simulink model "autopilot_total"  (R2021b)
settings: Solver=ode4  StartTime=0.0  StopTime=T  FixedStep=P.Ts  RelTol=1e-6  AbsTol=1e-3  EnableMultiTasking=on
values from neighbouring files (symbols this model uses):
  k_VI = 0.8    [forces_moments_testing.m]
  k_VP = 0.5    [forces_moments_testing.m]
undefined symbols (not defined in the file or in its folder): forces_moments, P, true_states
libraries: simulink x3
settings Model: Creator=beard  LastModifiedBy=joaomoura
settings SolverCC: AutoScaleAbsTol=off  AlgebraicLoopSolver=TrustRegion
settings DataIOCC: LimitDataPoints=on  SaveFormat=Array  ReturnWorkspaceOutputs=off
settings OptimizationCC: ExpressionDepthLimit=2147483647  InitFltsAndDblsToZero=on  LifeSpan=inf
settings DebuggingCC: UnderspecifiedInitializationDetection=Classic  MergeDetectMultiDrivingBlocksExec=none  SolverPrmCheckMsg=warning  FcnCallInpInsideContextMsg=warning  StateNameClashWarn=warning  PregeneratedLibrarySubsystemCodeDiagnostic=none  SFUnexpectedBacktrackingDiag=warning  SFNoUnconditionalDefaultTransitionDiag=warning  SFExecutionAtInitializationDiag=none  SFMachineParentedDataDiag=warning  ArithmeticOperatorsInVariantConditions=warning
settings HardwareCC: ProdBitPerPointer=32  ProdBitPerSizeT=32  ProdBitPerPtrDiffT=32  ProdLargestAtomicFloat=None  ProdIntDivRoundTo=Undefined  ProdEndianess=Unspecified  ProdWordSize=32  ProdHWDeviceType=32-bit Generic
settings ModelReferenceCC: PropagateSignalLabelsOutOfModel=off
settings SFSimCC: SimUseLocalCustomCode=off  CustomCodeUndefinedFunction=UseInterfaceOnly
settings RTWCC: RTWUseLocalCustomCode=off
settings CodeAppCC: StateflowObjectComments=on
settings GRTTargetCC: TargetLangStandard=C89/C90 (ANSI)  CombineOutputUpdateFcns=off  GRTInterface=on
settings ConfigComp: CovMetricSettings=dw  CovSaveCumulativeToWorkspaceVar=on  CovSaveSingleToWorkspaceVar=on  CovExternalEMLEnable=off  CovSFcnEnable=off

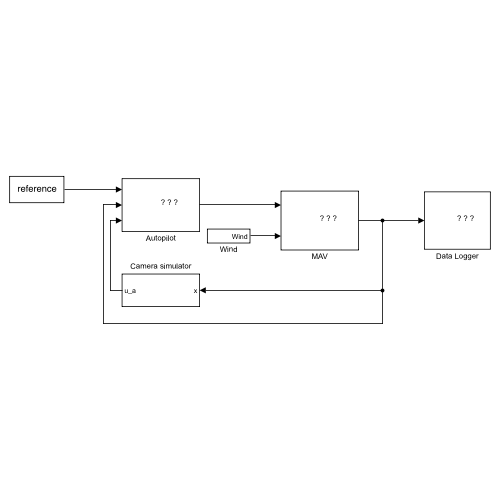
[thumbnail: Simulink's stored preview of the top-level diagram]
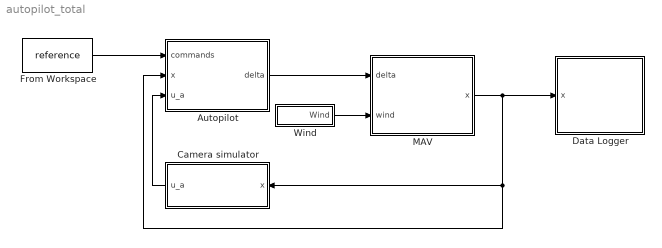
== system autopilot_total ==
  Autopilot : Subsystem
      mask Display: image(imread('simulink_imgs/kestrel.jpg'))
  Camera simulator : Subsystem
  Data Logger : Subsystem
      mask Display: image(imread('simulink_imgs/data_logger.png'))
  From Workspace : FromWorkspace  VariableName=reference
  MAV : Subsystem
      mask Display: image(imread('simulink_imgs/batcam.png'))
  Wind : Subsystem
  wires:
  Wind/1(Wind) -> MAV/2(wind)
  MAV/1(x) -> Camera simulator/1(x), Autopilot/2(x), Data Logger/1(x)
  Autopilot/1(delta) -> MAV/1(delta)
  From Workspace/1 -> Autopilot/1(commands)
  Camera simulator/1(u_a) -> Autopilot/3(u_a)

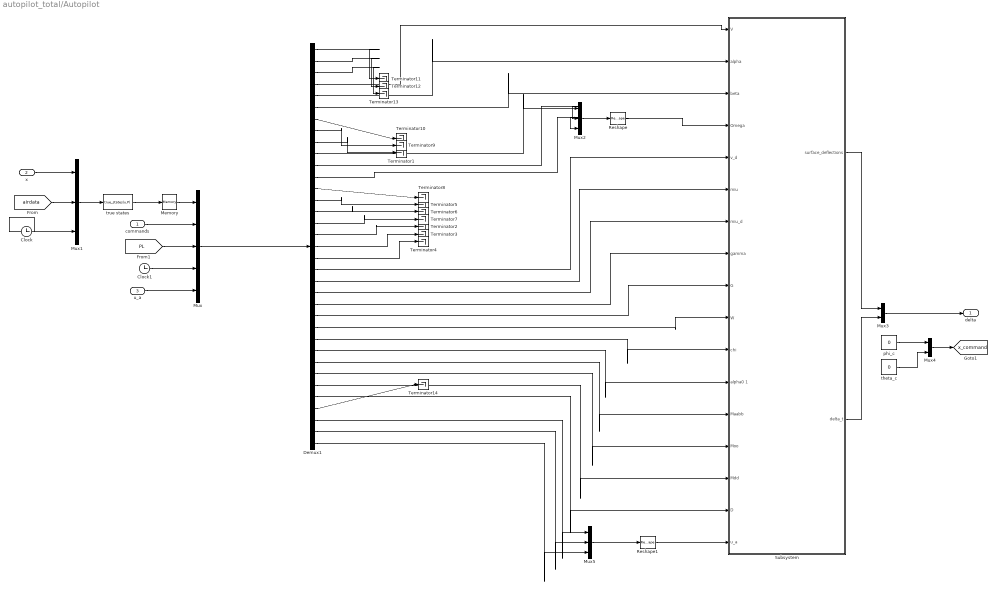
== system autopilot_total/Autopilot ==
  commands : Inport
  x : Inport  Port=2
  u_a : Inport  Port=3
  Clock : Clock
  Clock1 : Clock
  Demux1 : Demux  Outputs=19+1+11+1+3
  Memory : Memory
  Mux : Mux  Inputs=5
  Mux1 : Mux  Inputs=3
  Mux2 : Mux  Inputs=3
  Mux3 : Mux  Inputs=2
  Mux4 : Mux  Inputs=2
  Mux5 : Mux  Inputs=3
  Reshape : Reshape  OutputDimensionality=Customize  OutputDimensions=[3,1]
  Reshape1 : Reshape  OutputDimensionality=Customize  OutputDimensions=[3,1]
  Subsystem : Subsystem
  Terminator{1..14} (14 alike) : Terminator
  phi_c : Constant  Value=0
  theta_c : Constant  Value=0
  true states : MATLABFcn  MATLABFcn=true_states(u,P)  OutputDimensions=19  SampleTime=P.Ts
  delta : Outport  VectorParamsAs1DForOutWhenUnconnected=off
  tag scope: x_command=global
  wires:
  Clock/1 -> Mux1/3
  Mux3/1 -> delta/1
  Mux4/1 -> [x_command]
  commands/1 -> Mux/2
  Mux1/1 -> true states/1
  x/1 -> Mux1/1
  true states/1 -> Memory/1
  [airdata] -> Mux1/2
  Memory/1 -> Mux/1
  Clock1/1 -> Mux/4
  [PL] -> Mux/3
  Mux/1 -> Demux1/1
  Demux1/4 -> Subsystem/1(V)
  Demux1/5 -> Subsystem/2(alpha)
  Demux1/6 -> Subsystem/3(beta)
  Demux1/20 -> Subsystem/5(v_d)
  Demux1/10 -> Mux2/1
  Demux1/11 -> Mux2/2
  Demux1/12 -> Mux2/3
  Mux2/1 -> Reshape/1
  Demux1/21 -> Subsystem/6(miu)
  Demux1/22 -> Subsystem/7(miu_d)
  Demux1/23 -> Subsystem/8(gamma)
  Demux1/24 -> Subsystem/9(G)
  Demux1/25 -> Subsystem/10(W)
  u_a/1 -> Mux/5
  Demux1/26 -> Subsystem/11(chi)
  Demux1/27 -> Subsystem/12(alpha0 1)
  Demux1/28 -> Subsystem/13(Maabb)
  Demux1/29 -> Subsystem/14(Moo)
  Demux1/30 -> Subsystem/15(Mdd)
  Demux1/19 -> Terminator4/1
  Demux1/18 -> Terminator3/1
  Demux1/17 -> Terminator2/1
  Demux1/16 -> Terminator7/1
  Demux1/15 -> Terminator6/1
  Demux1/14 -> Terminator5/1
  Demux1/13 -> Terminator8/1
  Demux1/9 -> Terminator1/1
  Demux1/8 -> Terminator9/1
  Demux1/7 -> Terminator10/1
  Demux1/3 -> Terminator13/1
  Demux1/2 -> Terminator12/1
  Demux1/1 -> Terminator11/1
  Subsystem/1(surface_deflections) -> Mux3/1
  Subsystem/2("delta_t ") -> Mux3/2
  phi_c/1 -> Mux4/1
  theta_c/1 -> Mux4/2
  Demux1/31 -> Subsystem/16(D)
  Demux1/32 -> Terminator14/1
  Reshape/1 -> Subsystem/4("Omega ")
  Demux1/33 -> Mux5/1
  Demux1/34 -> Mux5/2
  Demux1/35 -> Mux5/3
  Mux5/1 -> Reshape1/1
  Reshape1/1 -> Subsystem/17(u_a)

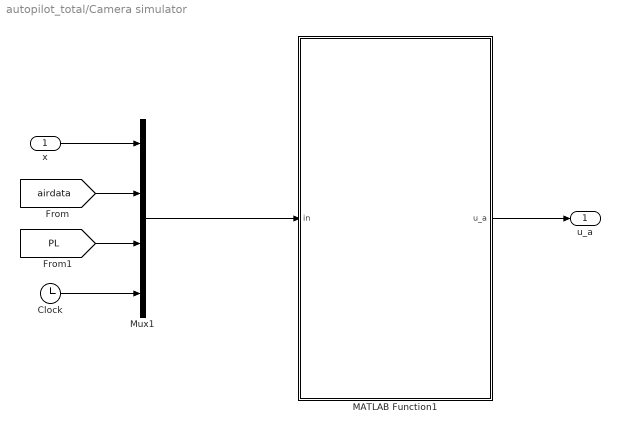
== system autopilot_total/Camera simulator ==
  x : Inport
  Clock : Clock
  MATLAB Function1 : MATLAB Function  TreatAsAtomicUnit=on
  Mux1 : Mux
  u_a : Outport
  wires:
  MATLAB Function1/1(u_a) -> u_a/1
  Clock/1 -> Mux1/4
  [airdata] -> Mux1/2
  [PL] -> Mux1/3
  Mux1/1 -> MATLAB Function1/1(in)
  x/1 -> Mux1/1

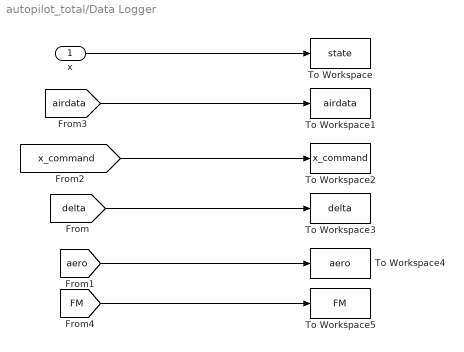
== system autopilot_total/Data Logger ==
  x : Inport
  To Workspace : ToWorkspace  VariableName=state  SaveFormat=Structure With Time  SampleTime=-1
  To Workspace1 : ToWorkspace  VariableName=airdata  SaveFormat=Structure With Time  SampleTime=-1
  To Workspace2 : ToWorkspace  VariableName=x_command  SaveFormat=Structure With Time  SampleTime=-1
  To Workspace3 : ToWorkspace  VariableName=delta  SaveFormat=Structure With Time  SampleTime=-1
  To Workspace4 : ToWorkspace  VariableName=aero  SaveFormat=Structure With Time  SampleTime=-1
  To Workspace5 : ToWorkspace  VariableName=FM  SaveFormat=Structure With Time  SampleTime=-1
  wires:
  x/1 -> To Workspace/1
  [x_command] -> To Workspace2/1
  [delta] -> To Workspace3/1
  [airdata] -> To Workspace1/1
  [aero] -> To Workspace4/1
  [FM] -> To Workspace5/1

== system autopilot_total/MAV ==
  note: Forces & Moments
  note: States
  delta : Inport
  wind : Inport  Port=2
  Dynamics : S-Function  FunctionName=mav_dynamics  Parameters=P  SFunctionDeploymentMode=off  EnableBusSupport=off
  Forces & Moments : Subsystem
  x : Outport  VectorParamsAs1DForOutWhenUnconnected=off
  tag scope: PL=global, airdata=global
  wires:
  Dynamics/1 -> Forces & Moments/1(x), x/1
  Forces & Moments/1("[F M]") -> Dynamics/1
  Forces & Moments/2(air data) -> [airdata]
  delta/1 -> Forces & Moments/2(delta)
  wind/1 -> Forces & Moments/3(wind)
  Forces & Moments/3(PL) -> [PL]

== system autopilot_total/Wind ==
  Constant2 : Constant  Value=[P.wind_n; P.wind_e; P.wind_d]
  Mux1 : Mux  Inputs=2
  Wind Gusts : Subsystem
  Wind : Outport  VectorParamsAs1DForOutWhenUnconnected=off
  wires:
  Constant2/1 -> Mux1/1
  Mux1/1 -> Wind/1
  Wind Gusts/1(gusts) -> Mux1/2

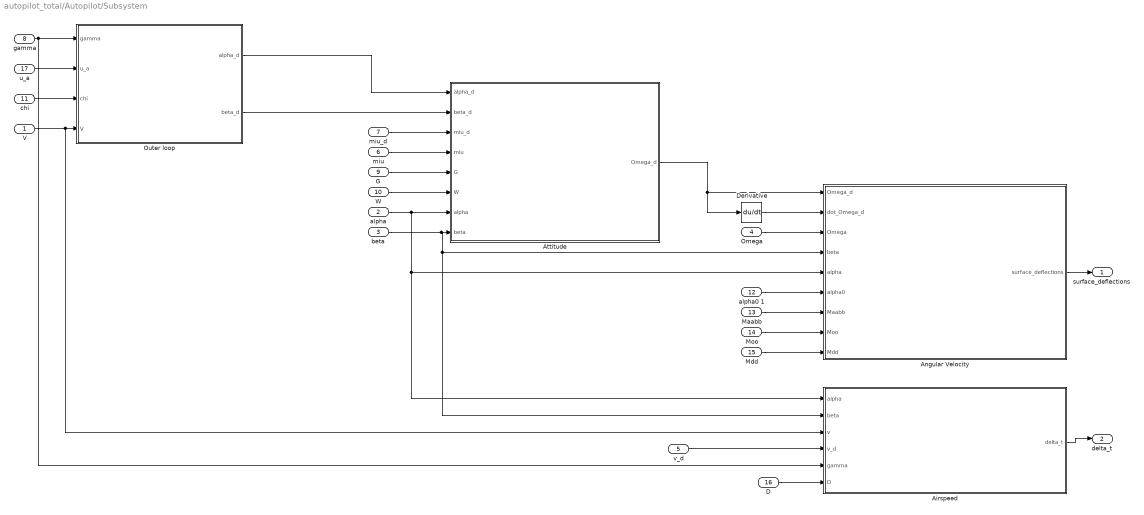
== system autopilot_total/Autopilot/Subsystem ==
  V : Inport
  alpha : Inport  Port=2
  beta : Inport  Port=3
  "Omega " : Inport  Port=4
  v_d : Inport  Port=5
  miu : Inport  Port=6
  miu_d : Inport  Port=7
  gamma : Inport  Port=8
  G : Inport  Port=9
  W : Inport  Port=10
  chi : Inport  Port=11
  alpha0 1 : Inport  Port=12
  Maabb : Inport  Port=13
  Moo : Inport  Port=14
  Mdd : Inport  Port=15
  D : Inport  Port=16
  u_a : Inport  Port=17
  Airspeed : Subsystem
  Angular Velocity : Subsystem
  Attitude : Subsystem
  Derivative : Derivative
  Outer loop : Subsystem
  surface_deflections : Outport  VectorParamsAs1DForOutWhenUnconnected=off
  "delta_t " : Outport  Port=2  VectorParamsAs1DForOutWhenUnconnected=off
  wires:
  Attitude/1(Omega_d) -> Derivative/1, Angular Velocity/1(Omega_d)
  Outer loop/2(beta_d) -> Attitude/2(beta_d)
  v_d/1 -> Airspeed/4(v_d)
  gamma/1 -> Outer loop/1(gamma), Airspeed/5(gamma)
  Airspeed/1("delta_t ") -> "delta_t "/1
  "Omega "/1 -> Angular Velocity/3(Omega)
  miu/1 -> Attitude/4(miu)
  beta/1 -> Airspeed/2(beta), Angular Velocity/4(beta), Attitude/8(beta)
  miu_d/1 -> Attitude/3(miu_d)
  Outer loop/1(alpha_d) -> Attitude/1(alpha_d)
  V/1 -> Outer loop/4(V), Airspeed/3("v ")
  Angular Velocity/1(surface_deflections) -> surface_deflections/1
  alpha/1 -> Attitude/7(alpha), Airspeed/1(alpha), Angular Velocity/5(alpha)
  u_a/1 -> Outer loop/2(u_a)
  chi/1 -> Outer loop/3(chi)
  Derivative/1 -> Angular Velocity/2(dot_Omega_d)
  G/1 -> Attitude/5(G)
  W/1 -> Attitude/6(W)
  alpha0 1/1 -> Angular Velocity/6(alpha0)
  Maabb/1 -> Angular Velocity/7(Maabb)
  Moo/1 -> Angular Velocity/8(Moo)
  Mdd/1 -> Angular Velocity/9(Mdd)
  D/1 -> Airspeed/6(D)

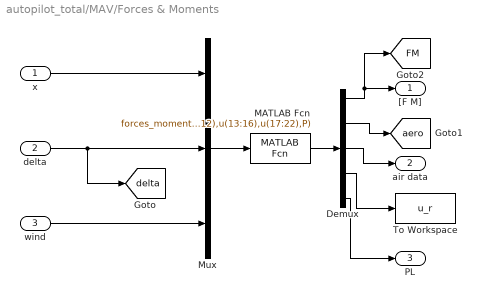
== system autopilot_total/MAV/Forces & Moments ==
  x : Inport
  delta : Inport  Port=2
  wind : Inport  Port=3
  Demux : Demux  Outputs=[6;6;6;1;11]
  MATLAB Fcn : MATLABFcn  MATLABFcn=forces_moments(u(1:12),u(13:16),u(17:22),P)  OutputDimensions=30
  Mux : Mux  Inputs=3
  To Workspace : ToWorkspace  VariableName=u_r  SampleTime=-1
  "[F M]" : Outport  VectorParamsAs1DForOutWhenUnconnected=off
  air data : Outport  Port=2  VectorParamsAs1DForOutWhenUnconnected=off
  PL : Outport  Port=3  VectorParamsAs1DForOutWhenUnconnected=off
  tag scope: FM=global, aero=global, delta=global
  wires:
  Mux/1 -> MATLAB Fcn/1
  Demux/1 -> [FM], "[F M]"/1
  MATLAB Fcn/1 -> Demux/1
  wind/1 -> Mux/3
  delta/1 -> Mux/2, [delta]
  x/1 -> Mux/1
  Demux/3 -> air data/1
  Demux/2 -> [aero]
  Demux/4 -> To Workspace/1
  Demux/5 -> PL/1

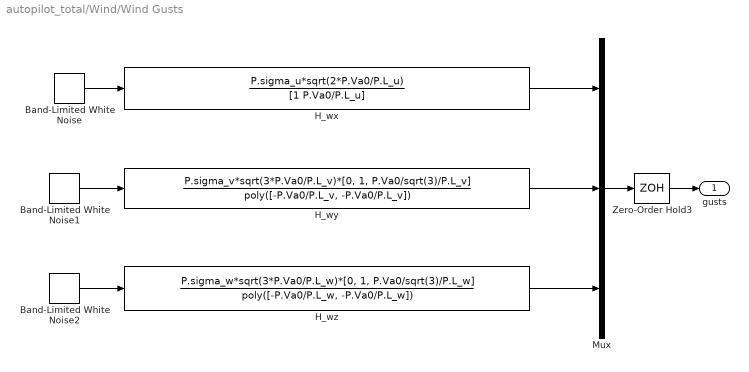
== system autopilot_total/Wind/Wind Gusts ==
  Band-Limited White Noise : simulink/Sources/Band-Limited White Noise  Cov=[1]  Ts=P.Ts  seed=[23341]
  Band-Limited White Noise1 : simulink/Sources/Band-Limited White Noise  Cov=[1]  Ts=P.Ts  seed=[23341]
  Band-Limited White Noise2 : simulink/Sources/Band-Limited White Noise  Cov=[1]  Ts=P.Ts  seed=[23341]
  H_wx : TransferFcn  Numerator=P.sigma_u*sqrt(2*P.Va0/P.L_u)  Denominator=[1 P.Va0/P.L_u]
  H_wy : TransferFcn  Numerator=P.sigma_v*sqrt(3*P.Va0/P.L_v)*[0, 1, P.Va0/sqrt(3)/P.L_v]  Denominator=poly([-P.Va0/P.L_v, -P.Va0/P.L_v])
  H_wz : TransferFcn  Numerator=P.sigma_w*sqrt(3*P.Va0/P.L_w)*[0, 1, P.Va0/sqrt(3)/P.L_w]  Denominator=poly([-P.Va0/P.L_w, -P.Va0/P.L_w])
  Mux : Mux  Inputs=3
  Zero-Order Hold3 : ZeroOrderHold  SampleTime=P.Ts
  gusts : Outport  VectorParamsAs1DForOutWhenUnconnected=off
  wires:
  H_wx/1 -> Mux/1
  Band-Limited White Noise/1 -> H_wx/1
  H_wy/1 -> Mux/2
  Band-Limited White Noise1/1 -> H_wy/1
  H_wz/1 -> Mux/3
  Band-Limited White Noise2/1 -> H_wz/1
  Mux/1 -> Zero-Order Hold3/1
  Zero-Order Hold3/1 -> gusts/1

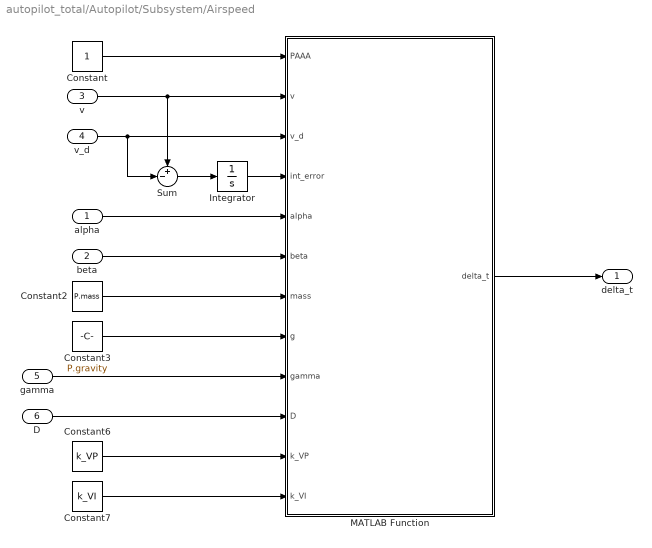
== system autopilot_total/Autopilot/Subsystem/Airspeed ==
  alpha : Inport
  beta : Inport  Port=2
  "v " : Inport  Port=3
  v_d : Inport  Port=4
  gamma : Inport  Port=5
  D : Inport  Port=6
  Constant : Constant
  Constant2 : Constant  Value=P.mass
  Constant3 : Constant  Value=P.gravity
  Constant6 : Constant  Value=k_VP
  Constant7 : Constant  Value=k_VI
  Integrator : Integrator
  MATLAB Function : MATLAB Function  TreatAsAtomicUnit=on
  Sum : Sum  Inputs=+-|
  "delta_t " : Outport  VectorParamsAs1DForOutWhenUnconnected=off
  wires:
  Constant3/1 -> MATLAB Function/8(g)
  gamma/1 -> MATLAB Function/9(gamma)
  Constant7/1 -> MATLAB Function/12(k_VI)
  beta/1 -> MATLAB Function/6(beta)
  Constant6/1 -> MATLAB Function/11(k_VP)
  MATLAB Function/1(delta_t) -> "delta_t "/1
  "v "/1 -> Sum/1, MATLAB Function/2(v)
  Integrator/1 -> MATLAB Function/4(int_error)
  alpha/1 -> MATLAB Function/5(alpha)
  Sum/1 -> Integrator/1
  Constant2/1 -> MATLAB Function/7(mass)
  Constant/1 -> MATLAB Function/1(PAAA)
  v_d/1 -> Sum/2, MATLAB Function/3(v_d)
  D/1 -> MATLAB Function/10(D)

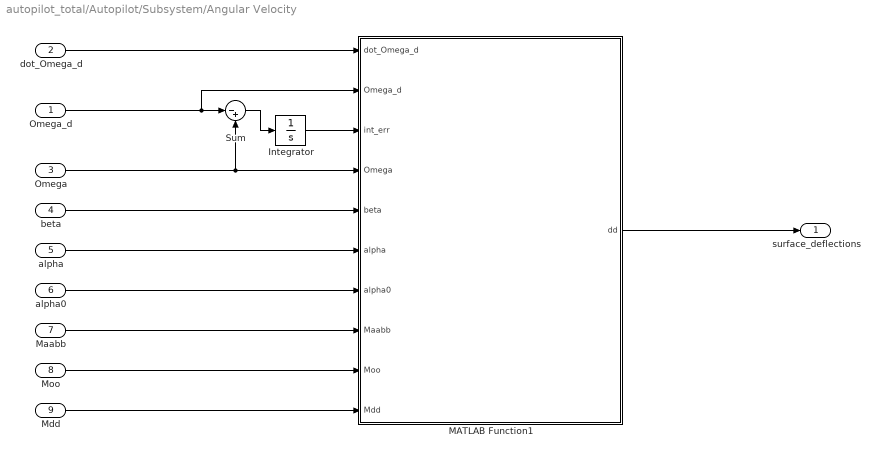
== system autopilot_total/Autopilot/Subsystem/Angular Velocity ==
  Omega_d : Inport
  dot_Omega_d : Inport  Port=2
  Omega : Inport  Port=3
  beta : Inport  Port=4
  alpha : Inport  Port=5
  alpha0 : Inport  Port=6
  Maabb : Inport  Port=7
  Moo : Inport  Port=8
  Mdd : Inport  Port=9
  Integrator : Integrator
  MATLAB Function1 : MATLAB Function  TreatAsAtomicUnit=on
  Sum : Sum  Inputs=|-+
  surface_deflections : Outport  VectorParamsAs1DForOutWhenUnconnected=off
  wires:
  Maabb/1 -> MATLAB Function1/8(Maabb)
  Omega_d/1 -> MATLAB Function1/2(Omega_d), Sum/1
  Sum/1 -> Integrator/1
  Mdd/1 -> MATLAB Function1/10(Mdd)
  dot_Omega_d/1 -> MATLAB Function1/1(dot_Omega_d)
  beta/1 -> MATLAB Function1/5(beta)
  Omega/1 -> Sum/2, MATLAB Function1/4(Omega)
  Moo/1 -> MATLAB Function1/9(Moo)
  alpha0/1 -> MATLAB Function1/7(alpha0)
  Integrator/1 -> MATLAB Function1/3(int_err)
  MATLAB Function1/1(dd) -> surface_deflections/1
  alpha/1 -> MATLAB Function1/6(alpha)

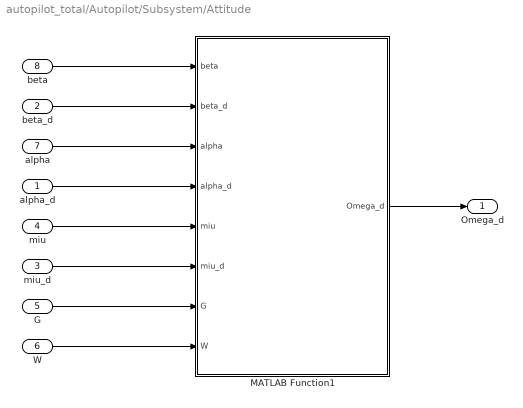
== system autopilot_total/Autopilot/Subsystem/Attitude ==
  alpha_d : Inport
  beta_d : Inport  Port=2
  miu_d : Inport  Port=3
  miu : Inport  Port=4
  G : Inport  Port=5
  W : Inport  Port=6
  alpha : Inport  Port=7
  beta : Inport  Port=8
  MATLAB Function1 : MATLAB Function  TreatAsAtomicUnit=on
  Omega_d : Outport  VectorParamsAs1DForOutWhenUnconnected=off
  wires:
  MATLAB Function1/1(Omega_d) -> Omega_d/1
  alpha_d/1 -> MATLAB Function1/4(alpha_d)
  beta_d/1 -> MATLAB Function1/2(beta_d)
  miu_d/1 -> MATLAB Function1/6(miu_d)
  miu/1 -> MATLAB Function1/5(miu)
  beta/1 -> MATLAB Function1/1(beta)
  alpha/1 -> MATLAB Function1/3(alpha)
  G/1 -> MATLAB Function1/7(G)
  W/1 -> MATLAB Function1/8(W)

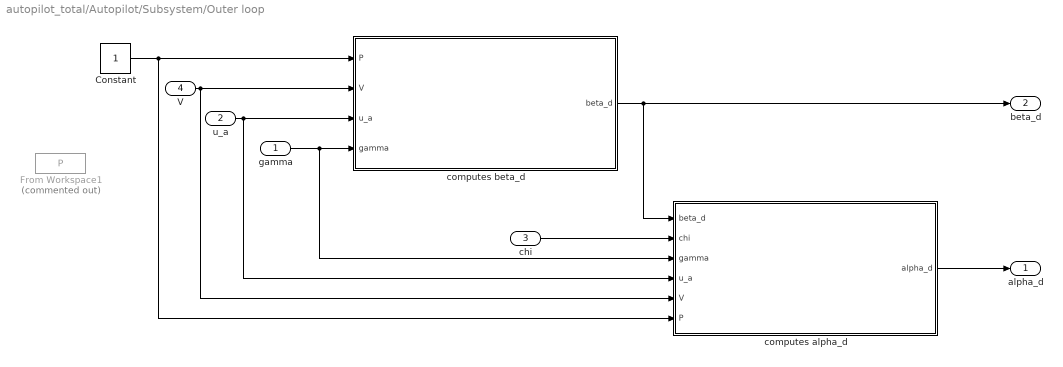
== system autopilot_total/Autopilot/Subsystem/Outer loop ==
  gamma : Inport
  u_a : Inport  Port=2
  chi : Inport  Port=3
  V : Inport  Port=4
  Constant : Constant
  From Workspace1 : FromWorkspace  Commented=on  VariableName=P
  computes alpha_d : Subsystem
  computes beta_d : Subsystem
  alpha_d : Outport
  beta_d : Outport  Port=2
  wires:
  computes beta_d/1(beta_d) -> computes alpha_d/1(beta_d), beta_d/1
  computes alpha_d/1(alpha_d) -> alpha_d/1
  gamma/1 -> computes alpha_d/3(gamma), computes beta_d/4(gamma)
  u_a/1 -> computes beta_d/3(u_a), computes alpha_d/4(u_a)
  chi/1 -> computes alpha_d/2(chi)
  Constant/1 -> computes alpha_d/6(P), computes beta_d/1(P)
  V/1 -> computes beta_d/2(V), computes alpha_d/5(V)

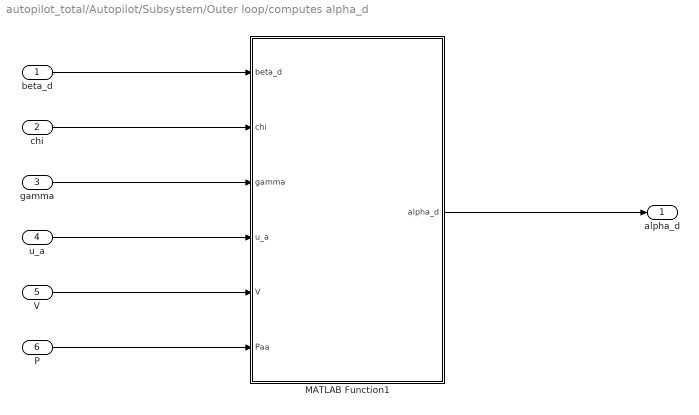
== system autopilot_total/Autopilot/Subsystem/Outer loop/computes alpha_d ==
  beta_d : Inport
  chi : Inport  Port=2
  gamma : Inport  Port=3
  u_a : Inport  Port=4
  V : Inport  Port=5
  P : Inport  Port=6
  MATLAB Function1 : MATLAB Function  TreatAsAtomicUnit=on
  alpha_d : Outport  VectorParamsAs1DForOutWhenUnconnected=off
  wires:
  MATLAB Function1/1(alpha_d) -> alpha_d/1
  beta_d/1 -> MATLAB Function1/1(beta_d)
  P/1 -> MATLAB Function1/6(Paa)
  u_a/1 -> MATLAB Function1/4(u_a)
  chi/1 -> MATLAB Function1/2(chi)
  gamma/1 -> MATLAB Function1/3(gamma)
  V/1 -> MATLAB Function1/5(V)

== system autopilot_total/Autopilot/Subsystem/Outer loop/computes beta_d ==
  P : Inport
  V : Inport  Port=2
  u_a : Inport  Port=3
  gamma : Inport  Port=4
  MATLAB Function1 : MATLAB Function  TreatAsAtomicUnit=on
  beta_d : Outport  VectorParamsAs1DForOutWhenUnconnected=off
  wires:
  MATLAB Function1/1(beta_d) -> beta_d/1
  P/1 -> MATLAB Function1/1(Paa)
  u_a/1 -> MATLAB Function1/3(u_a)
  gamma/1 -> MATLAB Function1/4(gamma)
  V/1 -> MATLAB Function1/2(V)

== matlab function autopilot_total/Autopilot/Subsystem/Outer loop/computes beta_d/MATLAB Function1 ==
  data: Paa input; V input; u_a input; gamma input; beta_d output
function beta_d = controller(Paa,V,u_a,gamma)
    P.mass = 25;
    P.rho = 1.2682;
    P.gravity = 9.8000;
    P.C_Y_beta = -0.9800;
    P.S_wing = 0.5500;
    
    % params
    q_bar = 0.5*P.rho*V^2;
    
    % control law

    beta_d = ([0;0;1]'*u_a*cos(gamma)) / (q_bar*P.S_wing*P.C_Y_beta - P.mass*P.gravity*sin(gamma));

end

== matlab function autopilot_total/Camera simulator/MATLAB Function1 ==
  data: in input; u_a output
% function u_a = ua(in)
%     % params
%     % vw is wind
%     
%     V = in(13);  
%     v = in(4,5,6); 
%     vw = [in(14,15),0];
% 
%     k1 = 1;
%     k3 = 5;
%     k4 = 3.5;
%     m = 25;
%     q = [1, 0, 0]; % Centroid                   %é só isto?
%     u = [0, 0 , 1]; % Direction of the lines    % duas vezes os mesmo u?
%     u = transpose([1, 0, 0]);
%     rho = transpose([0, 1, 0]);
%     n = transpose([0, 0, 1]);
%     delta1 = transpose(n)*q;
%     vwy = transpose(rho)*vw;
%     vdy = -k1*delta1 - vwy;
%     v = transpose(rho)*v;
%     d = -n*(v + vw);
%     w_star = 0.4; % desired translational optical flow in the direction n.
%     w = (v +vw)/d; 
%     vy = v(2);  % vy = transpose(rho)*
%     delta3 = vy - vdy;
%     % control law
% 
%     u_a = (m*V) / (transpose(v)*u)*(k1*k3*delta3*n-k4*(transpose(n)*w-w_star)*rho);
% 
% end

%function u_a = ua(n,rho, cam,points1,points2, vel, m, V, wind,u,k1,k3,k4, R)
%function u_a = ua(pos, vel, V, wind)
function u_a = ua(in)
    % assume cam = [x, y, z] where x, y and z are measured in relation to L
    % (0, 0 ,0) is the position of the camera assumed in the center of mass
    % of the aircraft
    % points1 - array with points of the left line
    % points2 - array with points of the right line
    % in this code it is assumed the points come in the following format:
    % points1 = [-5,0,0, -5,5,0, -5,10,0, -5,15,0]; % line on the left
    % wind = [wx, wy, wz]     
    % vel = [vx, vy, vz] of the plane relative to the wind
    % V the velocity of the aircraft
    % k1, k3 and k4 are gain values
    % m the mass
    % R is the rotation matrix
    L = [0,0,0];


    pos = [in(1),in(2),in(3)]';
    vel = [in(4),in(5),in(6)]';
    V = in(13);  
    wind = [in(14),in(15),0]';

    cam = [pos(1)- L(1), pos(2)- L(2), (-pos(3)) - L(3)]; %pos of aircraft relative to L


    k1 = 1;
    k3 = 5;
    k4 = 3.5;
    mass = 25;

    n = [0, 0, 1]';
    rho = [0, 1, 0]';
    u = [1, 0, 0]';

    points1 = [-5,0,0, -5,5,0, -5,10,0, -5,15,0];
    points2 = [5,0,0, 5,5,0, 5,10,0, 5,15,0];
    
    R = rotx(10);  %o que é aqui??

    P1 = reshape(points1, 3, floor(length(points1)/3))';
     % Assuming an ideal spherical camera
    q = [0 0 0];
    for i=1:floor(length(points1)/3)
        for j=1:floor(length(points1)/3)
            if j>i
                img1=P1(i,:)/norm(P1(i,:));
                img2=P1(j,:)/norm(P1(j,:));
                h = (cross(img1, img2))/norm(cross(img1, img2))*R;
                q = q + h;
            end
        end
    end
    P2 = reshape(points2, 3, floor(length(points2)/3))';
     for i=1:floor(length(points1)/3)
        for j=1:floor(length(points1)/3)
            if j>i
                img1=P2(i,:)/norm(P2(i,:));
                img2=P2(j,:)/norm(P2(j,:));
                h = (cross(img1, img2))/norm(cross(img1, img2))*R;
                q = q + h;
            end
        end
     end
    
    w_star = 0.4; % s^-1 desired translational optical flow in the direction n
    d = sqrt((cam(1))^2+(cam(2))^2+(cam(3))^2);
    tof = transpose(n)*(vel+wind)/d; % translational optical flow 
    delta1 = transpose(n)*(q-rho);
    vdy = -k1*delta1 - wind(2); 
    delta3 = vel(2) - vdy;
    % u_a calculation
    u_a = mass*V/(transpose(vel)*u)*(k1*k3*delta3*n-k4*(tof-w_star)*rho);

end

== matlab function autopilot_total/Autopilot/Subsystem/Airspeed/MATLAB Function ==
  data: PAAA input; v input; v_d input; delta_t output; int_error input; alpha input; beta input; mass input; g input; gamma input; D input; k_VP input; k_VI input
function delta_t = airspeedController(PAAA,v,v_d,int_error,alpha,beta,mass,g,gamma,D,k_VP,k_VI)
% Equation 47 [1]
    P.k_motor = 80;
    P.rho = 1.2682;
    P.S_prop = 0.2027;
    P.C_prop = 1;
    

    F_T = [(D + mass*g*sin(gamma))/(cos(beta)*cos(alpha))] + ...
        [(k_VP*(v-v_d) + k_VI*int_error)/(cos(beta)*cos(alpha))];

    delta_t = (1/P.k_motor)*sqrt((2*F_T/(P.rho*P.S_prop*P.C_prop)+v^2));
    
end



% gamma é a primeira cordenada do wing angle

% [1] Serra, Pedro & Cunha, Rita & Hamel, T. & Silvestre, Carlos & Le Bras, Florent. (2015). Nonlinear Image-Based Visual Servo Controller for the Flare Maneuver of Fixed-Wing Aircraft Using Optical Flow. IEEE Transactions on Control Systems Technology. 23. 570–583. 10.1109/TCST.2014.2330996.

== matlab function autopilot_total/Autopilot/Subsystem/Angular Velocity/MATLAB Function1 ==
  data: dot_Omega_d input; Omega_d input; int_err input; Omega input; beta input; alpha input; alpha0 input; Maabb input; dd output; Moo input; Mdd input
function dd = controller(dot_Omega_d,Omega_d,int_err,Omega,beta,alpha,alpha0,Maabb,Moo,Mdd)
% Equation 48 [1]

    % gains
    kp = 1;
    ki = 1;
    
    % auxiliary calculations
    Soo = skew(Omega);
    
    
    % control law
%     dd = Mdd^-1 *(Soo*eye(3)*Omega-...
%         Maabb*[beta;alpha-alpha0]-...
%         Moo*Omega-...
%         kp*(Omega-Omega_d)-...
%         ki*int_err+dot_Omega_d);

     dd = Mdd^-1 *(Soo*eye(3)*Omega- ...
        Moo*Omega-...
        kp*(Omega-Omega_d)-...
        ki*int_err+dot_Omega_d);
end

function S = skew(vector) 
    S = [0,-vector(3),vector(2);
        vector(3),0,-vector(1);
        -vector(2),vector(1),0];
end

% [1] Serra, Pedro & Cunha, Rita & Hamel, T. & Silvestre, Carlos & Le Bras, Florent. (2015). Nonlinear Image-Based Visual Servo Controller for the Flare Maneuver of Fixed-Wing Aircraft Using Optical Flow. IEEE Transactions on Control Systems Technology. 23. 570–583. 10.1109/TCST.2014.2330996.

== matlab function autopilot_total/Autopilot/Subsystem/Attitude/MATLAB Function1 ==
  data: beta input; beta_d input; alpha input; alpha_d input; miu input; miu_d input; G input; Omega_d output; W input
function Omega_d = controller(beta,beta_d,alpha,alpha_d,miu,miu_d,G,W)

    % gains
    Kp = 1;
    % control law
    Omega_d = G\(-W-Kp*[beta-beta_d;alpha-alpha_d;miu-miu_d]);
end

== matlab function autopilot_total/Autopilot/Subsystem/Outer loop/computes alpha_d/MATLAB Function1 ==
  data: beta_d input; chi input; gamma input; u_a input; V input; Paa input; alpha_d output
function alpha_d = controller(beta_d,chi,gamma,u_a,V,Paa)
    
    P.mass = 25;
    P.rho = 1.2682;
    P.C_D_alpha = 0.300;
    P.C_L_alpha = 3.4500;
    P.S_wing = 0.5500;
    P.C_D_0 = 0.0300;
    P.C_Y_beta = -0.980;
    P.gravity = 9.8000;
    P.C_L_0 = 0.2800;


    % params
    q_bar = 0.5*P.rho*V^2;

    ad1 = q_bar * P.S_wing * P.C_D_alpha;
    ad2 = q_bar * P.S_wing * (P.C_L_alpha + P.C_D_0 - P.C_Y_beta * beta_d * tan(beta_d))...
        + P.mass*P.gravity * sin(gamma) * 1/cos(beta_d);

    ad3 = -P.mass*P.gravity*cos(gamma) + q_bar*P.S_wing*P.C_L_0 - [0;1;0]' * u_a/cos(chi);

    % control law

    alpha_d = (-ad2 + sqrt(ad2^2-4*ad1*ad3))/(2*ad1);

end


% duvida: na equação no paper (ultima pagina) tem la: Cl0_linha e Cd0_linha
% e nao Cl0 e Cd0, no entanto não se fala mais desses parâmetros (com
% linha) no paper e nós também não temos isso e eu nao sei o que é
